simulink model "airspeed_pitch_loop"  (R2016a)
settings: Solver=VariableStepAuto  StartTime=0.0  StopTime=10.0  RelTol=1e-3
values from neighbouring files (symbols this model uses):
  a_V1 = 0.4039    [tune_arispeed_pitch.m]
  K_theta_DC = 0.4591    [tune_arispeed_pitch.m]
  v_ki = -wn_airspeed_pitch^2 / (K_theta_DC * 9.81)    (= -0.11204195986)    [tune_arispeed_pitch.m]
  v_kp = (a_V1-2*zeta_airspeed_pitch*wn_airspeed_pitch)/(K_theta_DC*0.81)    (= -1.61493915901)    [tune_arispeed_pitch.m]
settings Model: Creator=andreanv  LastModifiedBy=andreanv

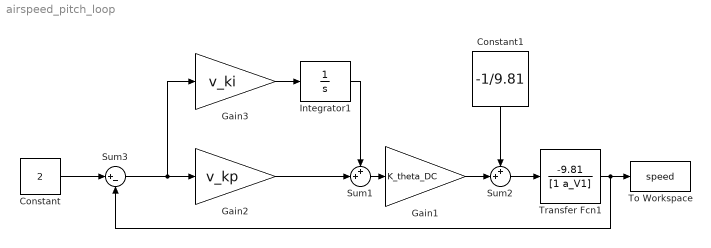
== system airspeed_pitch_loop ==
  Constant : Constant  Value=2
  Constant1 : Constant  Value=-1/9.81
  Gain1 : Gain  Gain=K_theta_DC
  Gain2 : Gain  Gain=v_kp
  Gain3 : Gain  Gain=v_ki
  Integrator1 : Integrator
  Sum1 : Sum  Inputs=++|
  Sum2 : Sum  Inputs=++|
  Sum3 : Sum  Inputs=|+-
  To Workspace : ToWorkspace  VariableName=speed  SaveFormat=Timeseries  SampleTime=-1
  Transfer Fcn1 : TransferFcn  Numerator=[-9.81]  Denominator=[1 a_V1]
  wires:
  Sum1/1 -> Gain1/1
  Sum2/1 -> Transfer Fcn1/1
  Transfer Fcn1/1 -> Sum3/2, To Workspace/1
  Gain2/1 -> Sum1/2
  Gain3/1 -> Integrator1/1
  Integrator1/1 -> Sum1/1
  Constant/1 -> Sum3/1
  Sum3/1 -> Gain3/1, Gain2/1
  Gain1/1 -> Sum2/2
  Constant1/1 -> Sum2/1
